simulink model "AdditionalPump_parallel"  (R2016b)
settings: Solver=ode45  StartTime=0.0  StopTime=200  MaxStep=5  RelTol=1e-3  EnableMultiTasking=on
undefined symbols (not defined in the file): path_carnot
libraries: carnot x8
settings Model: Creator=drhf  LastModifiedBy=drhf
settings DataIOCC: LimitDataPoints=on  SaveFormat=Array  SignalLoggingSaveFormat=ModelDataLogs
settings OptimizationCC: ExpressionDepthLimit=2147483647  LifeSpan=inf
settings DebuggingCC: UnderspecifiedInitializationDetection=Classic  MergeDetectMultiDrivingBlocksExec=none  SolverPrmCheckMsg=warning  StateNameClashWarn=warning  SFUnexpectedBacktrackingDiag=warning  SFNoUnconditionalDefaultTransitionDiag=warning  SFExecutionAtInitializationDiag=none
settings HardwareCC: ProdBitPerPointer=32  ProdBitPerSizeT=32  ProdBitPerPtrDiffT=32  ProdLargestAtomicFloat=None  ProdIntDivRoundTo=Undefined  ProdEndianess=Unspecified  ProdWordSize=32  ProdHWDeviceType=32-bit Generic
settings ModelReferenceCC: PropagateSignalLabelsOutOfModel=off
settings GRTTargetCC: TargetLangStandard=C89/C90 (ANSI)  GeneratePreprocessorConditionals=Disable all  CombineOutputUpdateFcns=off  GRTInterface=on
settings ConfigComp: CovMetricSettings=dw  CovHtmlReporting=on  CovSaveCumulativeToWorkspaceVar=on  CovSaveSingleToWorkspaceVar=on  CovExternalEMLEnable=off

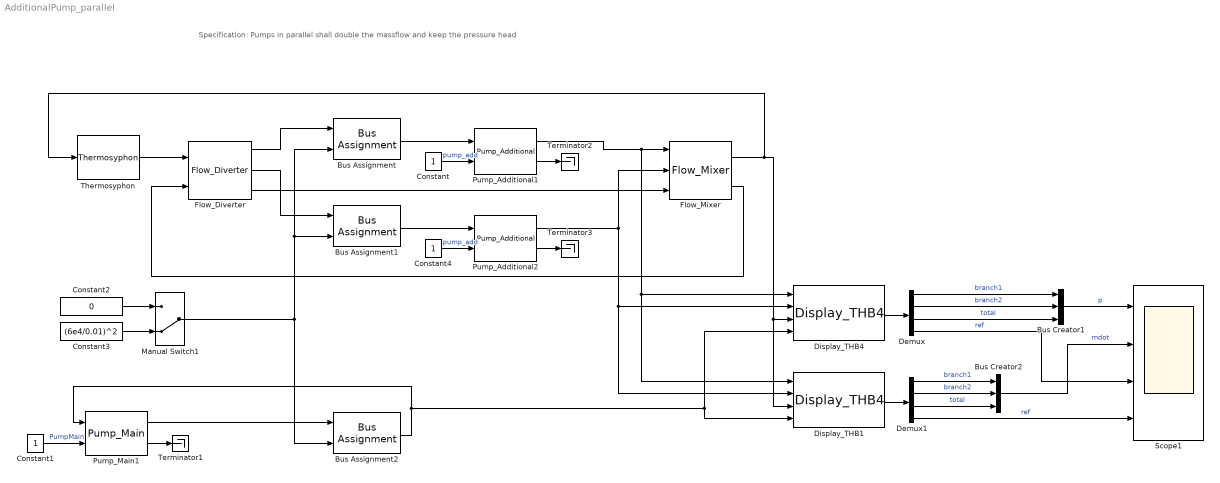
== system AdditionalPump_parallel ==
  note: Specification:
      | Pumps in parallel shall double the massflow and keep the pressure head
  Bus Assignment : BusAssignment  AssignedSignals=DPQuadratic
  Bus Assignment1 : BusAssignment  AssignedSignals=DPQuadratic
  Bus Assignment2 : BusAssignment  AssignedSignals=DPQuadratic
  Bus Creator1 : BusCreator  Inputs=3
  Bus Creator2 : BusCreator  Inputs=3
  Constant : Constant
  Constant1 : Constant
  Constant2 : Constant  Value=0
  Constant3 : Constant  Value=(6e4/0.01)^2
  Constant4 : Constant
  Demux : Demux
  Demux1 : Demux
  Display_THB1 : carnot/Outputs/Display_THB4  t=off  m=on  p=off  id=off  mix=off  d=off
  Display_THB4 : carnot/Outputs/Display_THB4  t=off  m=off  p=on  id=off  mix=off  d=off
  Flow_Diverter : carnot/Hydraulics/Flow_Diverter
  Flow_Mixer : carnot/Hydraulics/Flow_Mixer  t=1
  Manual Switch1 : ManualSwitch  CurrentSetting=0
  Pump_Additional1 : carnot/Hydraulics/Pump_Additional  Tini=20  PathName=fullfile(path_carnot('libsl'), 'Hydraulics', 'Pump_Main', 'parameter_set')  FileName='Pump6m.mat'  userPath=off  userParam=off  a0=60000  a1=-43200  a2=0  dia=0.025  UA=1  mcp=4182  e0=50  e1=28.8  e2=-10.368
  Pump_Additional2 : carnot/Hydraulics/Pump_Additional  Tini=20  PathName=fullfile(path_carnot('libsl'), 'Hydraulics', 'Pump_Main', 'parameter_set')  FileName='Pump6m.mat'  userPath=off  userParam=off  a0=60000  a1=-43200  a2=0  dia=0.025  UA=1  mcp=4182  e0=50  e1=28.8  e2=-10.368
  Pump_Main1 : carnot/Hydraulics/Pump_Main  Tini=20  p0=3e5  IDpreset=pressure drop  fluid=Water  mix=0  mix2=0  mix3=0  t1=0.1  PathName=fullfile(path_carnot('libsl'), 'Hydraulics', 'Pump_Main', 'parameter_set')  FileName='Pump6m.mat'  userPath=off  userParam=off  a0=60000  a1=-43200  a2=0  dia=0.025  UA=1  mcp=4182  e0=50  e1=28.8  e2=-10.368
  Scope1 : Scope  NumInputPorts=4
  Terminator1 : Terminator
  Terminator2 : Terminator
  Terminator3 : Terminator
  Thermosyphon : carnot/Hydraulics/Thermosyphon  dia=0.025  fluid_id=Water  mix=0  mix2=0  mix3=0  p0=3e5  t1=0.1
  wires:
  Pump_Additional1/2 -> Terminator2/1
  Constant1/1 -> Pump_Main1/2  "PumpMain"
  Bus Assignment/1 -> Pump_Additional1/1
  Display_THB4/1 -> Demux/1
  Demux/1 -> Bus Creator1/1  "branch1"
  Demux/2 -> Bus Creator1/2  "branch2"
  Demux/3 -> Bus Creator1/3  "total"
  Bus Creator1/1 -> Scope1/1  "p"
  Constant/1 -> Pump_Additional1/2  "pump_add"
  Pump_Main1/2 -> Terminator1/1
  Bus Assignment2/1 -> Pump_Main1/1, Display_THB4/4, Display_THB1/4
  Manual Switch1/1 -> Bus Assignment2/2, Bus Assignment1/2, Bus Assignment/2
  Bus Creator2/1 -> Scope1/2  "mdot"
  Thermosyphon/1 -> Flow_Diverter/1
  Pump_Main1/1 -> Bus Assignment2/1
  Constant2/1 -> Manual Switch1/1
  Constant3/1 -> Manual Switch1/2
  Pump_Additional2/2 -> Terminator3/1
  Bus Assignment1/1 -> Pump_Additional2/1
  Constant4/1 -> Pump_Additional2/2  "pump_add"
  Pump_Additional2/1 -> Display_THB1/2, Display_THB4/2, Flow_Mixer/2
  Flow_Diverter/1 -> Bus Assignment/1
  Flow_Diverter/2 -> Bus Assignment1/1
  Flow_Diverter/3 -> Flow_Mixer/3
  Pump_Additional1/1 -> Flow_Mixer/1, Display_THB4/1, Display_THB1/1
  Flow_Mixer/1 -> Display_THB1/3, Display_THB4/3, Thermosyphon/1
  Flow_Mixer/2 -> Flow_Diverter/2
  Demux/4 -> Scope1/3  "ref"
  Display_THB1/1 -> Demux1/1
  Demux1/1 -> Bus Creator2/1  "branch1"
  Demux1/2 -> Bus Creator2/2  "branch2"
  Demux1/3 -> Bus Creator2/3  "total"
  Demux1/4 -> Scope1/4  "ref"
